simulink model "untitled"  (R2015a)
settings: Solver=ode45  StartTime=0.0  StopTime=10  RelTol=1e-3
undefined symbols (not defined in the file or in its folder): C, L, R
settings Model: Creator=Amanda  LastModifiedBy=Amanda

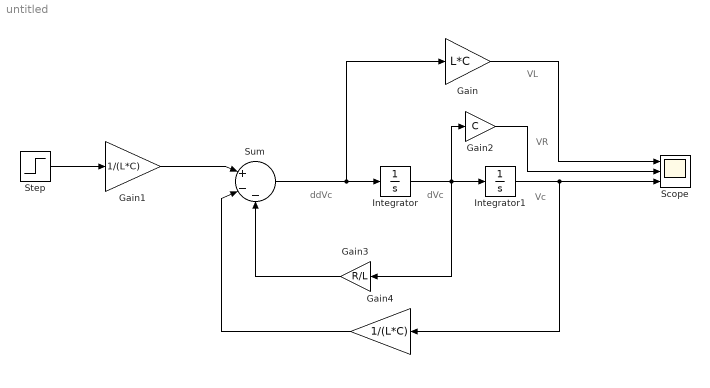
== system untitled ==
  note: Vc
  note: VR
  note: VL
  note: dVc
  note: ddVc
  Gain : Gain  Gain=L*C
  Gain1 : Gain  Gain=1/(L*C)
  Gain2 : Gain  Gain=C
  Gain3 : Gain  Gain=R/L
  Gain4 : Gain  Gain=1/(L*C)
  Integrator : Integrator
  Integrator1 : Integrator
  Scope : Scope  NumInputPorts=3
      settings: YMin=-5~-5~-5  YMax=5~5~5
  Step : Step  SampleTime=0
  Sum : Sum  Inputs=|+--
  wires:
  Sum/1 -> Integrator/1, Gain/1
  Step/1 -> Gain1/1
  Gain1/1 -> Sum/1
  Integrator/1 -> Gain3/1, Integrator1/1, Gain2/1
  Gain3/1 -> Sum/3
  Gain4/1 -> Sum/2
  Integrator1/1 -> Gain4/1, Scope/3
  Gain/1 -> Scope/1
  Gain2/1 -> Scope/2
